simulink model "labik10"  (R2022b)
settings: Solver=VariableStepAuto  StartTime=0.0  StopTime=10.0  RelTol=1e-3
undefined symbols (not defined in the file or in its folder): K, Tm, Tt
settings Model: Creator=micha  LastModifiedBy=mateu

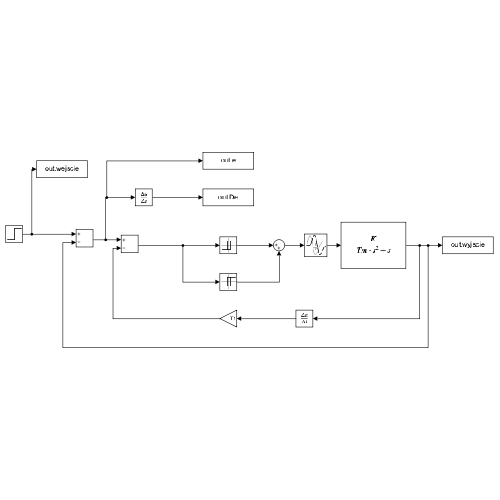
[thumbnail: Simulink's stored preview of the top-level diagram]
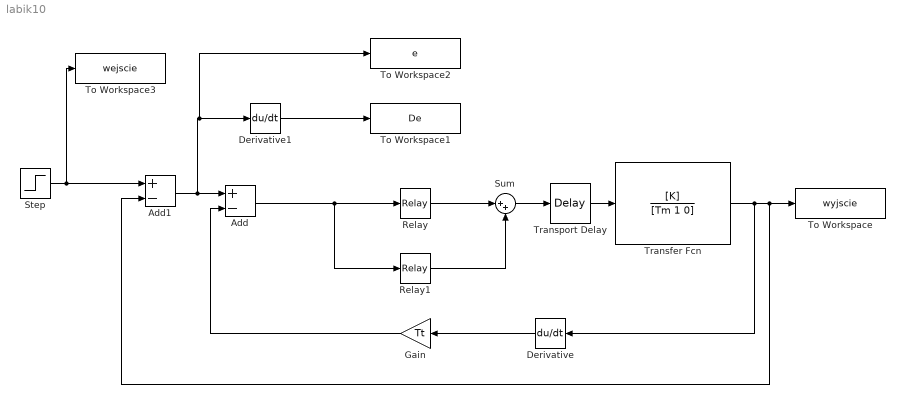
== system labik10 ==
  Add : Sum  Inputs=+-
  Add1 : Sum  Inputs=+-
  Derivative : Derivative
  Derivative1 : Derivative
  Gain : Gain  Gain=Tt
  Relay : Relay  OnSwitchValue=0.073  OffSwitchValue=0.05  OnOutputValue=3
  Relay1 : Relay  OnSwitchValue=-0.05  OffSwitchValue=-0.073  OnOutputValue=0  OffOutputValue=-3
  Step : Step  Time=0  SampleTime=0.1
  Sum : Sum  Inputs=|++
  To Workspace : ToWorkspace  VariableName=wyjscie  SampleTime=-1
  To Workspace1 : ToWorkspace  VariableName=De  SampleTime=-1
  To Workspace2 : ToWorkspace  VariableName=e  SampleTime=-1
  To Workspace3 : ToWorkspace  VariableName=wejscie  SampleTime=-1
  Transfer Fcn : TransferFcn  Numerator=[K]  Denominator=[Tm 1 0]
  Transport Delay : TransportDelay
  wires:
  Relay/1 -> Sum/1
  Add/1 -> Relay1/1, Relay/1
  Relay1/1 -> Sum/2
  Sum/1 -> Transport Delay/1
  Transport Delay/1 -> Transfer Fcn/1
  Transfer Fcn/1 -> Add1/2, To Workspace/1, Derivative/1
  Derivative/1 -> Gain/1
  Gain/1 -> Add/2
  Add1/1 -> To Workspace2/1, Derivative1/1, Add/1
  Step/1 -> To Workspace3/1, Add1/1
  Derivative1/1 -> To Workspace1/1
